simulink model "linearized_decoupling"  (R2016b)
settings: Solver=VariableStepAuto  StartTime=0.0  StopTime=10.0  RelTol=1e-3
values from neighbouring files (symbols this model uses):
  A = simplify(A)    [symbolic_rotor.m]
  B = B_dbth    [decoupling_falb_wolovich.m]    (also in symbolic_rotor.m = simplify(B))
  C = [0,0,0,-L*mg*cos(beta)*beta_dot;0,0,0,L*mg*sin(beta)*beta_dot;0,0,0,0;0,0,0,0]    [disturbance_compensation_nonlinear_test.m]    (also in symbolic_rotor.m = [1,0,0,0, 0,0,0,0; uav_grasp_opt.m = [0,0,L*mg*sin(theta)*theta_dot;0,0,L*mg*cos(theta)*theta_dot; uav_grasp_opt_var_mass.m)
  M = D_star\K    [decoupling_falb_wolovich.m]
  R = D_star\F    [decoupling_falb_wolovich.m]    (also in plot_rings_file.m = [u(1)^2*C+c, u(1)*u(2)*C-u(3)*s, u(1)*u(3)*C+u(2)*s; posvelacc_time_opt.m = [u(1)^2*C+c, u(1)*u(2)*C-u(3)*s, u(1)*u(3)*C+u(2)*s; riccati_controller_linear.m = diag([100,100,10]); uav_grasp_opt.m = diag([1;10]))
  x0 = zeros(8,1)    [decoupling_falb_wolovich.m]    (also in disturbance_compensation.m; disturbance_compensation_nonlinear_test.m = [0;0;0;pi/2;0;0;0;0]; riccati_controller_linear.m; symbolic_rotor.m)
settings Model: Creator=Administrator  LastModifiedBy=Administrator

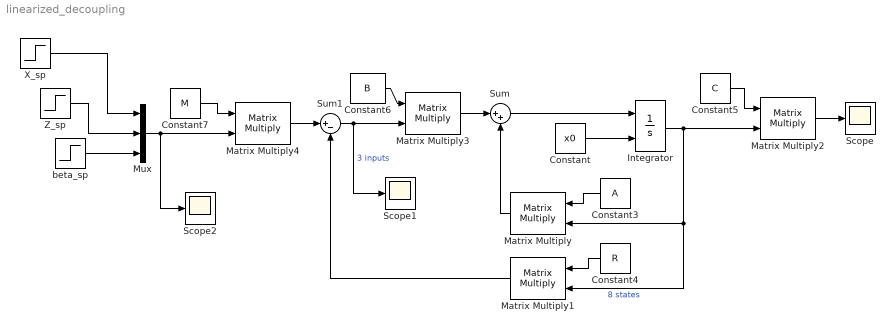
== system linearized_decoupling ==
  Constant : Constant  Value=x0
  Constant3 : Constant  Value=A
  Constant4 : Constant  Value=R
  Constant5 : Constant  Value=C
  Constant6 : Constant  Value=B
  Constant7 : Constant  Value=M
  Integrator : Integrator  InitialConditionSource=external
  Matrix Multiply{,1..4} (5 alike) : Product  Multiplication=Matrix(*)
  Mux : Mux  Inputs=3
  Scope : Scope
  Scope1 : Scope
  Scope2 : Scope
  Sum : Sum  Inputs=|++
  Sum1 : Sum  Inputs=|+-
  X_sp : Step  SampleTime=0  VectorParams1D=off
  Z_sp : Step  SampleTime=0  VectorParams1D=off
  beta_sp : Step  Time=6  After=0.3  SampleTime=0  VectorParams1D=off
  wires:
  Constant/1 -> Integrator/2
  Sum/1 -> Integrator/1
  Integrator/1 -> Matrix Multiply1/2, Matrix Multiply/2, Matrix Multiply2/2  "8 states"
  Matrix Multiply/1 -> Sum/2
  Matrix Multiply3/1 -> Sum/1
  Matrix Multiply1/1 -> Sum1/2
  Matrix Multiply4/1 -> Sum1/1
  Matrix Multiply2/1 -> Scope/1
  Constant3/1 -> Matrix Multiply/1
  Mux/1 -> Scope2/1, Matrix Multiply4/2
  Constant7/1 -> Matrix Multiply4/1
  Constant6/1 -> Matrix Multiply3/1
  Sum1/1 -> Scope1/1, Matrix Multiply3/2  "3 inputs"
  Constant4/1 -> Matrix Multiply1/1
  Constant5/1 -> Matrix Multiply2/1
  X_sp/1 -> Mux/1
  Z_sp/1 -> Mux/2
  beta_sp/1 -> Mux/3
